simulink model "sampleModel321"  (R2021b)
settings: Solver=VariableStepAuto  StartTime=0.0  StopTime=10.0  RelTol=1e-3
undefined symbols (not defined in the file or in its folder): DiscIntNeverNeededParam, Newton, Raphson
libraries: simulink x5, slpidlib x3
settings Model: Creator=user  LastModifiedBy=user

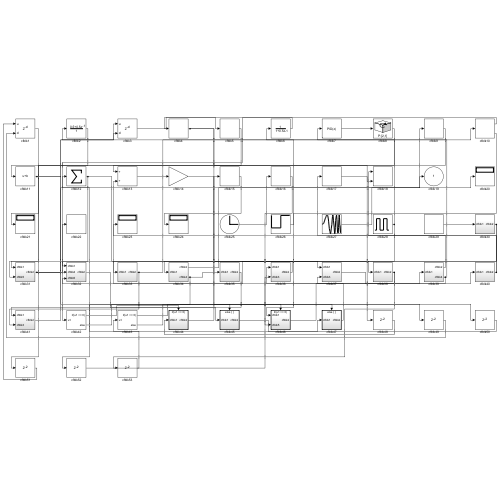
[thumbnail: Simulink's stored preview of the top-level diagram]
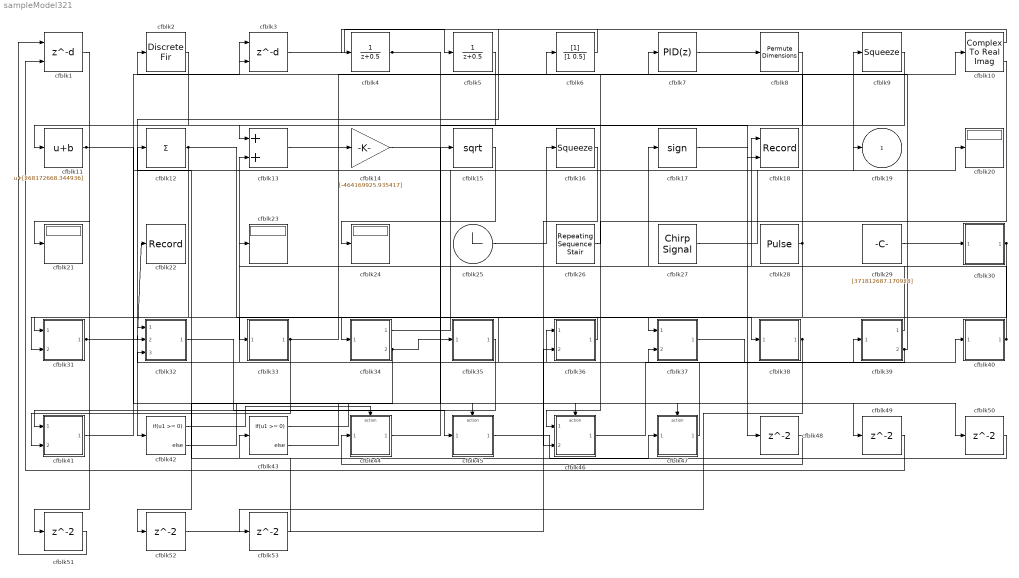
== system sampleModel321 ==
  cfblk1 : Delay  DelayLengthSource=Input port  SampleTime=1
      settings: InputPortMap=u0,p1
  cfblk10 : ComplexToRealImag
  cfblk11 : Bias  Bias=[268172668.344936]
  cfblk12 : Sum  Inputs=+
  cfblk13 : Sum
  cfblk14 : Gain  Gain=[-464169925.935417]
  cfblk15 : Sqrt  SaturateOnIntegerOverflow=on
  cfblk16 : Squeeze
  cfblk17 : Signum
  cfblk18 : Record  FileSettingsInternal="{\"entries\":[{\"content\":{\"excelSettings\":{\"content\":{},\"type\":\"Streamout.ExcelSettings\"}},\"type\":\"Streamout.FileSettingStorage\",\"uuid\":\"425e636b-3fce-4782-b074-d740fdb3f4d9\"}],\"packageUris\":[\"http://schema.mathworks.com/mf0/streamout_blocks/R2020a\"],\"version\":\"1.0\"}"  Layout=[1 1]  SignalsInternal="{\"entries\":[{\"content\":{\"signals\":[{\"content\":{\"blockPath\":[\"sampleModel321/cfblk18\"],\"channel\":[],\"dimensions\":[1,1],\"domain\":\"sampleModel321/cfblk18\",\"lineColor\":\"#a2142f\",\"plots\":[1],\"port\":1,\"sid\":[\"\"],\"signalID\":13570,\"signalName\":\"cfblk39:1\"},\"type\":\"RecordBlkView.Signal\",\"uuid\":\"76a65c16-e679-48b2-815a-f076962d0f51\"},{\"content\":{\"blockPath\":[\"sampleModel321/cfblk18\"],\"channel\":[],\"dimensions\":[1],\"domain\":\"sampleModel321/cfblk18\",\"lineColor\":\"#139fff\",\"plots\":[1],\"port\":2,\"sid\":[\"\"],\"signalID\":13574,\"signalName\":\"cfblk4\"},\"type\":\"RecordBlkView.Signal\",\"uuid\":\"fd042eb1-360a-48a8-a6a7-0b4ece49d86c\"}]},\"type\":\"RecordBlkView.InputSignals\",\"uuid\":\"04defab3-50e2-434c-8494-9e9e2b3fbd45\"}],\"packageUris\":[\"http://schema.mathworks.com/mf0/streamout_blocks/R2020a\"],\"version\":\"1.0\"}"  VisualizationBindings="{\"xyplotplugin\":{\"info\":[{\"series\":[{\"bindingParametersList\":[{\"parameter\":\"X-Axis\",\"signalID\":13570,\"signalName\":\"cfblk39:1\"},{\"parameter\":\"Y-Axis\",\"signalID\":13574,\"signalName\":\"cfblk4\"}],\"seriesID\":37804}],\"subplotID\":1}]}}"  CompatibilityTag=XY
  cfblk2 : DiscreteFir  SampleTime=1
  cfblk{20..21,23..24} (4 alike) : Display
  cfblk22 : Record  FileSettingsInternal="{\"entries\":[{\"content\":{\"excelSettings\":{\"content\":{},\"type\":\"Streamout.ExcelSettings\"}},\"type\":\"Streamout.FileSettingStorage\",\"uuid\":\"e5cb3130-8903-4eb8-9594-fc3a84093773\"}],\"packageUris\":[\"http://schema.mathworks.com/mf0/streamout_blocks/R2020a\"],\"version\":\"1.0\"}"  SignalsInternal="{\"entries\":[{\"content\":{\"signals\":[{\"content\":{\"blockPath\":[\"sampleModel321/cfblk22\"],\"channel\":[],\"dimensions\":[1],\"domain\":\"sampleModel321/cfblk22\",\"lineColor\":\"#64d413\",\"plots\":[1],\"port\":1,\"sid\":[\"\"],\"signalID\":13578,\"signalName\":\"cfblk31\"},\"type\":\"RecordBlkView.Signal\",\"uuid\":\"8d54b6ac-4730-4698-b009-edcb357c7c86\"}]},\"type\":\"RecordBlkView.InputSignals\",\"uuid\":\"1d945891-151d-430b-b5ea-9e2fbc47fabc\"}],\"packageUris\":[\"http://schema.mathworks.com/mf0/streamout_blocks/R2020a\"],\"version\":\"1.0\"}"  VisualizationBindings="{\"sparklinesplugin\":{\"info\":[{\"bindingParametersList\":[],\"subplotID\":1}]}}"
  cfblk25 : Clock
  cfblk26 : simulink/Sources/Repeating Sequence Stair  OutValues=[386250561.955697, 569774263.015907]  tsamp=-1  OutMin=[]  OutMax=[]  OutDataTypeStr=double  OutputDataTypeScalingMode=double  OutDataType=fixdt(0,8)  ConRadixGroup=Best Precision: Vector-wise  OutScaling=2^-12
  cfblk27 : simulink/Sources/Chirp Signal  f1=[602586507.739925]  T=[637953242.487700]  f2=[388026924.623615]
  cfblk28 : DiscretePulseGenerator  PulseType=Time based  Amplitude=[932501065.133908]  Period=[39885667.681772]  PulseWidth=5  PhaseDelay=[8.000000]
  cfblk29 : Constant  Value=[371812687.170928]  SampleTime=1
  cfblk3 : Delay  DelayLengthSource=Input port  SampleTime=1
      settings: InputPortMap=u0,p1
  cfblk30 : Subsystem
  cfblk31 : Subsystem
  cfblk32 : Subsystem
  cfblk33 : Subsystem
  cfblk34 : Subsystem
  cfblk35 : Subsystem
  cfblk36 : Subsystem
  cfblk37 : Subsystem
  cfblk38 : Subsystem
  cfblk39 : Subsystem
  cfblk4 : DiscreteTransferFcn  SampleTime=1
  cfblk40 : Subsystem
  cfblk41 : Subsystem
  cfblk42 : If  IfExpression=u1 >= 0  SampleTime=1
  cfblk43 : If  IfExpression=u1 >= 0  SampleTime=1
  cfblk44 : Subsystem  TreatAsAtomicUnit=on
  cfblk45 : Subsystem  TreatAsAtomicUnit=on
  cfblk46 : Subsystem  TreatAsAtomicUnit=on
  cfblk47 : Subsystem  TreatAsAtomicUnit=on
  cfblk{48..53} (6 alike) : Delay  SampleTime=1
  cfblk5 : DiscreteTransferFcn  SampleTime=1
  cfblk6 : DiscreteFilter  SampleTime=1
  cfblk7 : slpidlib/PID Controller  Controller=PID  Form=Parallel  TimeDomain=Discrete-time  UseExternalTs=off  SampleTime=1  IntegratorMethod=Forward Euler  FilterMethod=Forward Euler  ControllerParametersSource=internal  P=1  I=1  D=0  UseFilter=on  N=100  TunerSelectOption=Transfer Function Based (PID Tuner App)  InitialConditionSource=internal  InitialConditionForIntegrator=0  InitialConditionForFilter=0  DifferentiatorICPrevScaledInput=0  ExternalReset=none  TrackingMode=off  Kt=1  LimitOutput=off  SatLimitsSource=internal  UpperSaturationLimit=inf  LowerSaturationLimit=-inf  LinearizeAsGain=off  AntiWindupMode=none  Kb=1  POutMin=[]  POutMax=[]  IOutMin=[]  IOutMax=[]  DOutMin=[]  DOutMax=[]  NOutMin=[]  NOutMax=[]  SumOutMin=[]  SumOutMax=[]  SaturationOutMin=[]  SaturationOutMax=[]  PParamMin=[]  PParamMax=[]  IParamMin=[]  IParamMax=[]  DParamMin=[]  DParamMax=[]  NParamMin=[]  NParamMax=[]  KbParamMin=[]  KbParamMax=[]  KtParamMin=[]  KtParamMax=[]  KbOutMin=[]  KbOutMax=[]  KtOutMin=[]  KtOutMax=[]  IntegratorOutMin=[]  IntegratorOutMax=[]  FilterOutMin=[]  FilterOutMax=[]  SumI1OutMin=[]  SumI1OutMax=[]  SumI2OutMin=[]  SumI2OutMax=[]  SumI3OutMin=[]  SumI3OutMax=[]  SumI4OutMin=[]  SumI4OutMax=[]  SumDOutMin=[]  SumDOutMax=[]  DifferentiatorOutMin=[]  DifferentiatorOutMax=[]  FilterDiffOutCoefMin=[]  FilterDiffOutCoefMax=[]  ReciprocalOutMin=[]  ReciprocalOutMax=[]  SumDenOutMin=[]  SumDenOutMax=[]  SumNumOutMin=[]  SumNumOutMax=[]  DivideOutMin=[]  DivideOutMax=[]  UdiffTsProdOutMin=[]  UdiffTsProdOutMax=[]  NTsProdOutMin=[]  NTsProdOutMax=[]  UintegralTsProdOutMin=[]  UintegralTsProdOutMax=[]  UngainTsProdOutMin=[]  UngainTsProdOutMax=[]  IntegratorContinuousStateAttributes=''  IntegratorStateMustResolveToSignalObject=off  IntegratorRTWStateStorageClass=Auto  FilterContinuousStateAttributes=''  FilterStateMustResolveToSignalObject=off  FilterRTWStateStorageClass=Auto  ParallelPVariant=InternalParameters  IdealPVariant=Disabled  IVariant=InternalParameters  DVariant=InternalParameters  IntegratorVariant=Discrete  SatVariant=Disabled  AWVariant=Passthrough  PCopyVariant=Disabled  TRVariant=Disabled  FdbkBlocksVariant=Forward  IdealPFdbkVariant=Disabled  SatFdbkVariant=Disabled  DerivativeFilterVariant=ForwardEulerFilter  NVariant=InternalParameters  NCopyVariant=Disabled  FilterICVariant=InternalICsFilter  IntegratorICVariant=InternalICs  ExternalResetVariant=Disabled  TRSumVariant=Passthrough  SumFdbkVariant=Disabled  SumVariant=Sum_PID  TsampFilterVariant=InternalTs  TsampNgainVariant=Passthrough  TsampIntegralVariant=Passthrough  ExternalSaturationOutDataTypeStr=Inherit: Same as second input
  cfblk8 : PermuteDimensions
  cfblk9 : Squeeze
  cfblk19 : Outport
  wires:
  cfblk8/1 -> cfblk13/1
  cfblk3/1 -> cfblk5/1
  cfblk47/1(cfblk2) -> cfblk36/1(cfblk1)
  cfblk34/1(cfblk2) -> cfblk9/1
  cfblk25/1 -> cfblk16/1
  cfblk30/1(cfblk2) -> cfblk13/2, cfblk31/2(cfblk5)
  cfblk10/1 -> cfblk42/1
  cfblk34/2(cfblk4) -> cfblk35/1(cfblk1), cfblk52/1
  cfblk28/1 -> cfblk2/1, cfblk33/1(cfblk1)
  cfblk12/1 -> cfblk38/1(cfblk1), cfblk32/1(cfblk1)
  cfblk29/1 -> cfblk30/1(cfblk1)
  cfblk41/1(cfblk2) -> cfblk19/1
  cfblk32/1(cfblk2) -> cfblk45/1(cfblk1)
  cfblk38/1(cfblk2) -> cfblk32/3(cfblk5), cfblk53/1
  cfblk9/1 -> cfblk11/1
  cfblk44/1(cfblk2) -> cfblk15/1
  cfblk26/1 -> cfblk6/1
  cfblk40/1(cfblk2) -> cfblk17/1, cfblk23/1
  cfblk13/1 -> cfblk14/1
  cfblk7/1 -> cfblk8/1
  cfblk1/1 -> cfblk31/1(cfblk1)
  cfblk15/1 -> cfblk24/1
  cfblk45/1(cfblk2) -> cfblk47/1(cfblk1)
  cfblk36/1(cfblk2) -> cfblk34/1(cfblk1)
  cfblk37/1(cfblk2) -> cfblk40/1(cfblk1)
  cfblk6/1 -> cfblk4/1
  cfblk27/1 -> cfblk20/1
  cfblk39/1(cfblk2) -> cfblk18/1
  cfblk10/2 -> cfblk46/1(cfblk1)
  cfblk31/1(cfblk2) -> cfblk22/1, cfblk32/2(cfblk4), cfblk3/1
  cfblk33/1(cfblk2) -> cfblk10/1, cfblk41/2(cfblk3)
  cfblk4/1 -> cfblk37/1(cfblk1), cfblk18/2
  cfblk16/1 -> cfblk46/2(cfblk5)
  cfblk35/1(cfblk2) -> cfblk41/1(cfblk1)
  cfblk39/2(cfblk4) -> cfblk37/2(cfblk3), cfblk7/1
  cfblk2/1 -> cfblk21/1
  cfblk11/1 -> cfblk3/2, cfblk50/1
  cfblk46/1(cfblk2) -> cfblk39/1(cfblk1)
  cfblk42/1 -> cfblk44/Action
  cfblk42/2 -> cfblk45/Action
  cfblk43/1 -> cfblk46/Action
  cfblk43/2 -> cfblk47/Action
  cfblk17/1 -> cfblk48/1
  cfblk48/1 -> cfblk44/1(cfblk1)
  cfblk14/1 -> cfblk49/1
  cfblk49/1 -> cfblk1/2
  cfblk50/1 -> cfblk43/1
  cfblk5/1 -> cfblk51/1
  cfblk51/1 -> cfblk1/1
  cfblk52/1 -> cfblk36/2(cfblk3)
  cfblk53/1 -> cfblk12/1

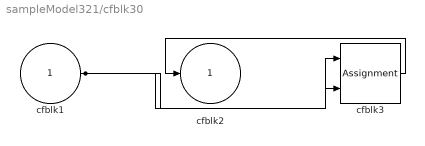
== system sampleModel321/cfblk30 ==
  cfblk1 : Inport
  cfblk3 : Assignment  DiagnosticForDimensions=Warning  IndexOptions=Index vector (dialog)  Indices=1  OutputSizes=1
  cfblk2 : Outport
  wires:
  cfblk3/1 -> cfblk2/1
  cfblk1/1 -> cfblk3/1, cfblk3/2

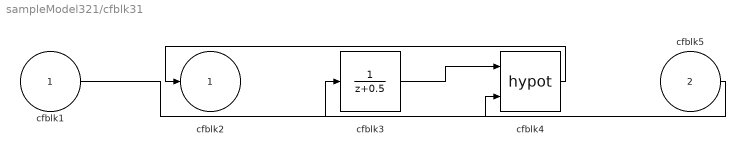
== system sampleModel321/cfblk31 ==
  cfblk1 : Inport
  cfblk5 : Inport  Port=2
  cfblk3 : DiscreteTransferFcn  SampleTime=1
  cfblk4 : Math  Operator=hypot  SaturateOnIntegerOverflow=on
  cfblk2 : Outport
  wires:
  cfblk4/1 -> cfblk2/1
  cfblk5/1 -> cfblk3/1
  cfblk3/1 -> cfblk4/1
  cfblk1/1 -> cfblk4/2

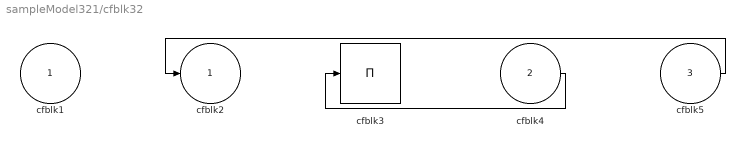
== system sampleModel321/cfblk32 ==
  cfblk1 : Inport
  cfblk4 : Inport  Port=2
  cfblk5 : Inport  Port=3
  cfblk3 : Product  Inputs=*
  cfblk2 : Outport
  wires:
  cfblk5/1 -> cfblk2/1
  cfblk4/1 -> cfblk3/1

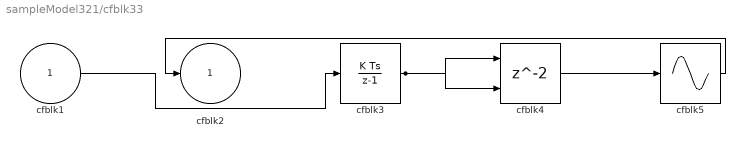
== system sampleModel321/cfblk33 ==
  cfblk1 : Inport
  cfblk3 : DiscreteIntegrator  ICPrevOutput=DiscIntNeverNeededParam  ICPrevScaledInput=DiscIntNeverNeededParam
  cfblk4 : Delay  ShowEnablePort=on  SampleTime=1
      settings: InputPortMap=u0,e6
  cfblk5 : Sin  TimeSource=Use external signal  SampleTime=0
  cfblk2 : Outport
  wires:
  cfblk5/1 -> cfblk2/1
  cfblk3/1 -> cfblk4/1, cfblk4/2
  cfblk1/1 -> cfblk3/1
  cfblk4/1 -> cfblk5/1

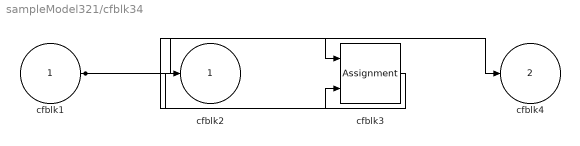
== system sampleModel321/cfblk34 ==
  cfblk1 : Inport
  cfblk3 : Assignment  DiagnosticForDimensions=Warning  IndexOptions=Index vector (dialog)  Indices=1  OutputSizes=1
  cfblk2 : Outport
  cfblk4 : Outport  Port=2
  wires:
  cfblk1/1 -> cfblk3/1, cfblk4/1, cfblk3/2
  cfblk3/1 -> cfblk2/1

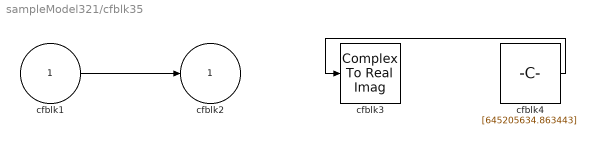
== system sampleModel321/cfblk35 ==
  cfblk1 : Inport
  cfblk3 : ComplexToRealImag
  cfblk4 : Constant  Value=[645205634.863443]  SampleTime=1
  cfblk2 : Outport
  wires:
  cfblk4/1 -> cfblk3/1
  cfblk1/1 -> cfblk2/1

== system sampleModel321/cfblk36 ==
  cfblk1 : Inport
  cfblk3 : Inport  Port=2
  cfblk2 : Outport
  wires:
  cfblk1/1 -> cfblk2/1

== system sampleModel321/cfblk37 ==
  cfblk1 : Inport
  cfblk3 : Inport  Port=2
  cfblk2 : Outport
  wires:
  cfblk1/1 -> cfblk2/1

== system sampleModel321/cfblk38 ==
  cfblk1 : Inport
  cfblk3 : Sqrt  Operator=rSqrt  AlgorithmType=Newton-Raphson  SaturateOnIntegerOverflow=on
  cfblk2 : Outport
  wires:
  cfblk1/1 -> cfblk3/1
  cfblk3/1 -> cfblk2/1

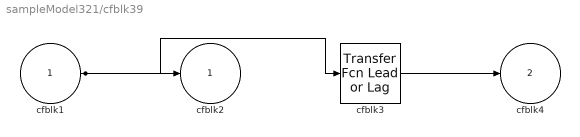
== system sampleModel321/cfblk39 ==
  cfblk1 : Inport
  cfblk3 : simulink/Discrete/Transfer Fcn Lead or Lag  PoleZ=0.95  ZeroZ=0.75  ICPrevOutput=0.0  ICPrevInput=0.0  DoSatur=off
      settings: SourceProductBaseCode=SL
  cfblk2 : Outport
  cfblk4 : Outport  Port=2
  wires:
  cfblk3/1 -> cfblk4/1
  cfblk1/1 -> cfblk2/1, cfblk3/1

== system sampleModel321/cfblk40 ==
  cfblk1 : Inport
  cfblk3 : Abs
  cfblk2 : Outport
  wires:
  cfblk3/1 -> cfblk2/1
  cfblk1/1 -> cfblk3/1

== system sampleModel321/cfblk41 ==
  cfblk1 : Inport
  cfblk3 : Inport  Port=2
  cfblk2 : Outport
  wires:
  cfblk1/1 -> cfblk2/1

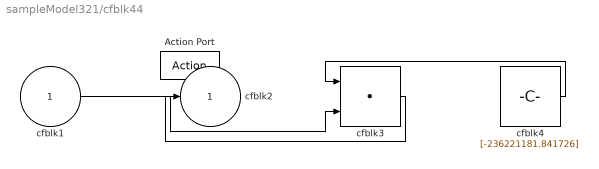
== system sampleModel321/cfblk44 ==
  cfblk1 : Inport
  Action Port : ActionPort  ActionPortLabel=if(u1 >= 0)
  cfblk3 : DotProduct  InputSameDT=on  OutDataTypeStr=Inherit: Inherit via internal rule
  cfblk4 : Constant  Value=[-236221181.841726]  SampleTime=1
  cfblk2 : Outport
  wires:
  cfblk4/1 -> cfblk3/1
  cfblk1/1 -> cfblk3/2
  cfblk3/1 -> cfblk2/1

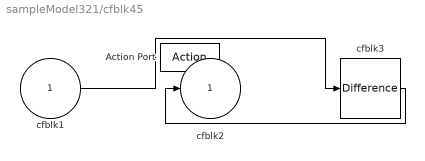
== system sampleModel321/cfblk45 ==
  cfblk1 : Inport
  Action Port : ActionPort  ActionPortLabel=else
  cfblk3 : simulink/Discrete/Difference  ICPrevInput=0.0  OutMin=[]  OutMax=[]  OutDataTypeStr=Inherit: Inherit via back propagation  OutDataType=fixdt(1, 16)  OutScaling=2^-10  DoSatur=off
  cfblk2 : Outport
  wires:
  cfblk3/1 -> cfblk2/1
  cfblk1/1 -> cfblk3/1

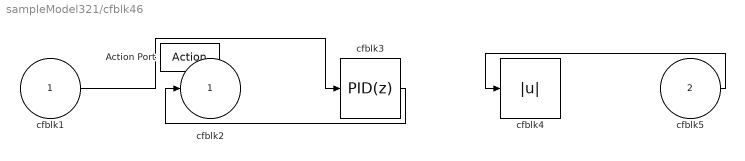
== system sampleModel321/cfblk46 ==
  cfblk1 : Inport
  cfblk5 : Inport  Port=2
  Action Port : ActionPort  ActionPortLabel=if(u1 >= 0)
  cfblk3 : slpidlib/PID Controller  Controller=PID  Form=Parallel  TimeDomain=Discrete-time  UseExternalTs=off  SampleTime=-1  IntegratorMethod=Forward Euler  FilterMethod=Forward Euler  ControllerParametersSource=internal  P=1  I=1  D=0  UseFilter=on  N=100  TunerSelectOption=Transfer Function Based (PID Tuner App)  InitialConditionSource=internal  InitialConditionForIntegrator=0  InitialConditionForFilter=0  DifferentiatorICPrevScaledInput=0  ExternalReset=none  TrackingMode=off  Kt=1  LimitOutput=off  SatLimitsSource=internal  UpperSaturationLimit=inf  LowerSaturationLimit=-inf  LinearizeAsGain=off  AntiWindupMode=none  Kb=1  POutMin=[]  POutMax=[]  IOutMin=[]  IOutMax=[]  DOutMin=[]  DOutMax=[]  NOutMin=[]  NOutMax=[]  SumOutMin=[]  SumOutMax=[]  SaturationOutMin=[]  SaturationOutMax=[]  PParamMin=[]  PParamMax=[]  IParamMin=[]  IParamMax=[]  DParamMin=[]  DParamMax=[]  NParamMin=[]  NParamMax=[]  KbParamMin=[]  KbParamMax=[]  KtParamMin=[]  KtParamMax=[]  KbOutMin=[]  KbOutMax=[]  KtOutMin=[]  KtOutMax=[]  IntegratorOutMin=[]  IntegratorOutMax=[]  FilterOutMin=[]  FilterOutMax=[]  SumI1OutMin=[]  SumI1OutMax=[]  SumI2OutMin=[]  SumI2OutMax=[]  SumI3OutMin=[]  SumI3OutMax=[]  SumI4OutMin=[]  SumI4OutMax=[]  SumDOutMin=[]  SumDOutMax=[]  DifferentiatorOutMin=[]  DifferentiatorOutMax=[]  FilterDiffOutCoefMin=[]  FilterDiffOutCoefMax=[]  ReciprocalOutMin=[]  ReciprocalOutMax=[]  SumDenOutMin=[]  SumDenOutMax=[]  SumNumOutMin=[]  SumNumOutMax=[]  DivideOutMin=[]  DivideOutMax=[]  UdiffTsProdOutMin=[]  UdiffTsProdOutMax=[]  NTsProdOutMin=[]  NTsProdOutMax=[]  UintegralTsProdOutMin=[]  UintegralTsProdOutMax=[]  UngainTsProdOutMin=[]  UngainTsProdOutMax=[]  IntegratorContinuousStateAttributes=''  IntegratorStateMustResolveToSignalObject=off  IntegratorRTWStateStorageClass=Auto  FilterContinuousStateAttributes=''  FilterStateMustResolveToSignalObject=off  FilterRTWStateStorageClass=Auto  ParallelPVariant=InternalParameters  IdealPVariant=Disabled  IVariant=InternalParameters  DVariant=InternalParameters  IntegratorVariant=Discrete  SatVariant=Disabled  AWVariant=Passthrough  PCopyVariant=Disabled  TRVariant=Disabled  FdbkBlocksVariant=Forward  IdealPFdbkVariant=Disabled  SatFdbkVariant=Disabled  DerivativeFilterVariant=ForwardEulerFilter  NVariant=InternalParameters  NCopyVariant=Disabled  FilterICVariant=InternalICsFilter  IntegratorICVariant=InternalICs  ExternalResetVariant=Disabled  TRSumVariant=Passthrough  SumFdbkVariant=Disabled  SumVariant=Sum_PID  TsampFilterVariant=InternalTs  TsampNgainVariant=Passthrough  TsampIntegralVariant=Passthrough  ExternalSaturationOutDataTypeStr=Inherit: Same as second input
  cfblk4 : Abs
  cfblk2 : Outport
  wires:
  cfblk3/1 -> cfblk2/1
  cfblk1/1 -> cfblk3/1
  cfblk5/1 -> cfblk4/1

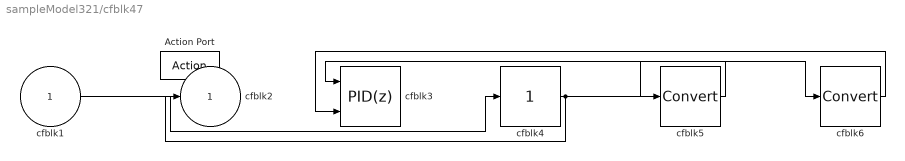
== system sampleModel321/cfblk47 ==
  cfblk1 : Inport
  Action Port : ActionPort  ActionPortLabel=else
  cfblk3 : slpidlib/PID Controller (2DOF)  Controller=PID  Form=Parallel  TimeDomain=Discrete-time  UseExternalTs=off  SampleTime=-1  IntegratorMethod=Forward Euler  FilterMethod=Forward Euler  ControllerParametersSource=internal  P=1  I=1  D=0  UseFilter=on  N=100  b=1  c=1  TunerSelectOption=Transfer Function Based (PID Tuner App)  InitialConditionSource=internal  InitialConditionForIntegrator=0  InitialConditionForFilter=0  DifferentiatorICPrevScaledInput=0  ExternalReset=none  TrackingMode=off  Kt=1  LimitOutput=off  SatLimitsSource=internal  UpperSaturationLimit=inf  LowerSaturationLimit=-inf  LinearizeAsGain=off  AntiWindupMode=none  Kb=1  POutMin=[]  POutMax=[]  IOutMin=[]  IOutMax=[]  DOutMin=[]  DOutMax=[]  NOutMin=[]  NOutMax=[]  bOutMin=[]  bOutMax=[]  cOutMin=[]  cOutMax=[]  SumOutMin=[]  SumOutMax=[]  SaturationOutMin=[]  SaturationOutMax=[]  PParamMin=[]  PParamMax=[]  IParamMin=[]  IParamMax=[]  DParamMin=[]  DParamMax=[]  NParamMin=[]  NParamMax=[]  bParamMin=[]  bParamMax=[]  cParamMin=[]  cParamMax=[]  KbParamMin=[]  KbParamMax=[]  KtParamMin=[]  KtParamMax=[]  KbOutMin=[]  KbOutMax=[]  KtOutMin=[]  KtOutMax=[]  IntegratorOutMin=[]  IntegratorOutMax=[]  FilterOutMin=[]  FilterOutMax=[]  SumI1OutMin=[]  SumI1OutMax=[]  SumI2OutMin=[]  SumI2OutMax=[]  SumI3OutMin=[]  SumI3OutMax=[]  SumI4OutMin=[]  SumI4OutMax=[]  SumDOutMin=[]  SumDOutMax=[]  Sum1OutMin=[]  Sum1OutMax=[]  Sum2OutMin=[]  Sum2OutMax=[]  Sum3OutMin=[]  Sum3OutMax=[]  DifferentiatorOutMin=[]  DifferentiatorOutMax=[]  FilterDiffOutCoefMin=[]  FilterDiffOutCoefMax=[]  ReciprocalOutMin=[]  ReciprocalOutMax=[]  SumDenOutMin=[]  SumDenOutMax=[]  SumNumOutMin=[]  SumNumOutMax=[]  DivideOutMin=[]  DivideOutMax=[]  UdiffTsProdOutMin=[]  UdiffTsProdOutMax=[]  NTsProdOutMin=[]  NTsProdOutMax=[]  UintegralTsProdOutMin=[]  UintegralTsProdOutMax=[]  UngainTsProdOutMin=[]  UngainTsProdOutMax=[]  IntegratorContinuousStateAttributes=''  IntegratorStateMustResolveToSignalObject=off  IntegratorRTWStateStorageClass=Auto  FilterContinuousStateAttributes=''  FilterStateMustResolveToSignalObject=off  FilterRTWStateStorageClass=Auto  ParallelPVariant=InternalParameters  IdealPVariant=Disabled  IVariant=InternalParameters  DVariant=InternalParameters  bVariant=InternalParameters  cVariant=InternalParameters  IntegratorVariant=Discrete  SatVariant=Disabled  AWVariant=Passthrough  PCopyVariant=Disabled  TRVariant=Disabled  FdbkBlocksVariant=Forward  IdealPFdbkVariant=Disabled  SatFdbkVariant=Disabled  DerivativeFilterVariant=ForwardEulerFilter  NVariant=InternalParameters  NCopyVariant=Disabled  FilterICVariant=InternalICsFilter  IntegratorICVariant=InternalICs  ExternalResetVariant=Disabled  TRSumVariant=Passthrough  SumFdbkVariant=Disabled  SumVariant=Sum_PID  TsampFilterVariant=InternalTs  TsampNgainVariant=Passthrough  TsampIntegralVariant=Passthrough  ExternalSaturationOutDataTypeStr=Inherit: Same as second input
      settings: SourceProductBaseCode=SL
  cfblk4 : simulink/Math Operations/Slider Gain  gain=1  low=0  high=2
  cfblk5 : DataTypeConversion
  cfblk6 : DataTypeConversion
  cfblk2 : Outport
  wires:
  cfblk1/1 -> cfblk4/1
  cfblk4/1 -> cfblk2/1, cfblk5/1, cfblk6/1
  cfblk5/1 -> cfblk3/1
  cfblk6/1 -> cfblk3/2
